simulink model "fuel_cell_tank"  (R2023a)
settings: Solver=VariableStepAuto  StartTime=0.0  StopTime=50  RelTol=1e-3
libraries: simulink x1
settings Model: Creator=connl  LastModifiedBy=connl

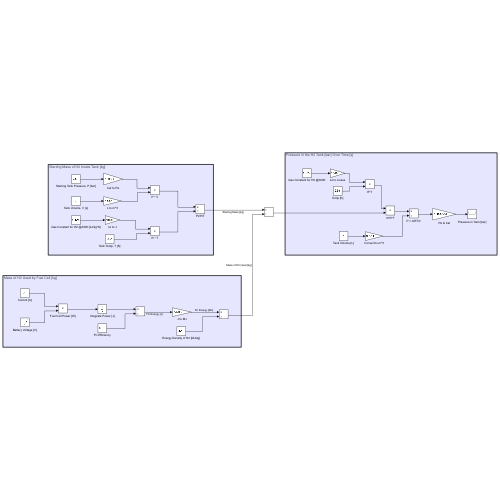
[thumbnail: Simulink's stored preview of the top-level diagram]
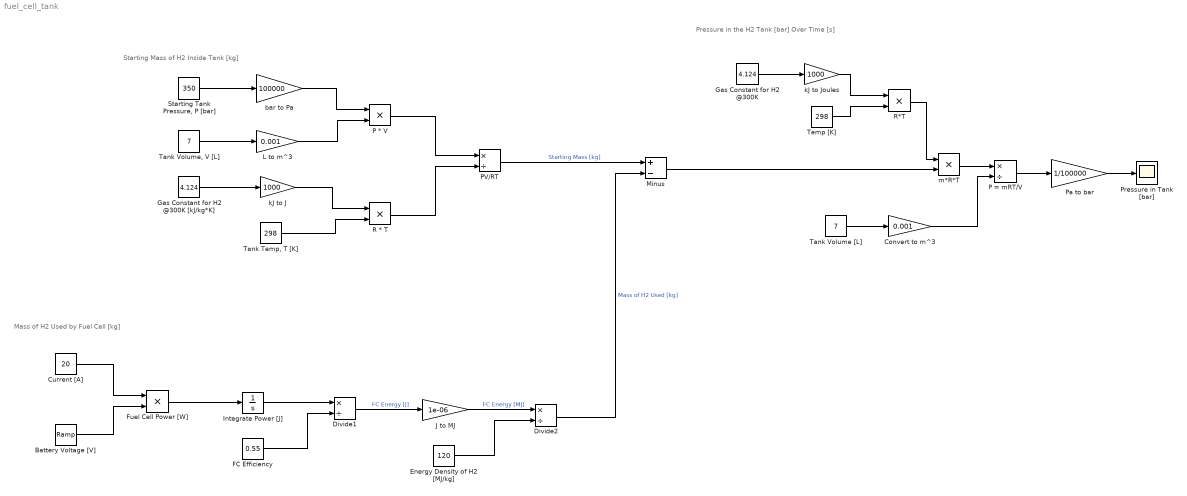
== system fuel_cell_tank ==
  note: Pressure in the H2 Tank [bar] Over Time [s]
  note: Mass of H2 Used by Fuel Cell [kg]
  note: Starting Mass of H2 Inside Tank [kg]
  Battery Voltage [V] : simulink/Sources/Ramp  slope=-1  start=0  InitialOutput=50
  Convert to m^3 : Gain  Gain=0.001
  Current [A] : Constant  Value=20
  Divide1 : Product  Inputs=*/
  Divide2 : Product  Inputs=*/
  Energy Density of H2 [MJ/kg] : Constant  Value=120
  FC Efficiency : Constant  Value=0.55
  Fuel Cell Power [W] : Product
  Gas Constant for H2 @300K : Constant  Value=4.124
  Gas Constant for H2 @300K [kJ/kg*K] : Constant  Value=4.124
  Integrate Power [J] : Integrator
  J to MJ : Gain  Gain=1e-06
  L to m^3 : Gain  Gain=0.001
  Minus : Sum  Inputs=+-
  P * V : Product
  P = mRT/V : Product  Inputs=*/
  PV/RT : Product  Inputs=*/
  Pa to bar : Gain  Gain=1/100000
  Pressure in Tank [bar] : Scope
  R * T : Product
  R*T : Product
  "Starting Tank Pressure, P [bar]" : Constant  Value=350
  "Tank Temp, T [K]" : Constant  Value=298
  Tank Volume [L] : Constant  Value=7
  "Tank Volume, V [L]" : Constant  Value=7
  Temp [K] : Constant  Value=298
  bar to Pa : Gain  Gain=100000
  kJ to J : Gain  Gain=1000
  kJ to Joules : Gain  Gain=1000
  m*R*T : Product
  wires:
  Integrate Power [J]/1 -> Divide1/1
  Divide2/1 -> Minus/2  "Mass of H2 Used [kg]"
  Fuel Cell Power [W]/1 -> Integrate Power [J]/1
  Current [A]/1 -> Fuel Cell Power [W]/1
  Battery Voltage [V]/1 -> Fuel Cell Power [W]/2
  Divide1/1 -> J to MJ/1  "FC Energy [J]"
  J to MJ/1 -> Divide2/1  "FC Energy [MJ]"
  bar to Pa/1 -> P * V/1
  FC Efficiency/1 -> Divide1/2
  Energy Density of H2 [MJ/kg]/1 -> Divide2/2
  "Starting Tank Pressure, P [bar]"/1 -> bar to Pa/1
  "Tank Volume, V [L]"/1 -> L to m^3/1
  L to m^3/1 -> P * V/2
  P * V/1 -> PV/RT/1
  "Tank Temp, T [K]"/1 -> R * T/2
  R * T/1 -> PV/RT/2
  Gas Constant for H2 @300K [kJ/kg*K]/1 -> kJ to J/1
  kJ to J/1 -> R * T/1
  PV/RT/1 -> Minus/1  "Starting Mass [kg]"
  Minus/1 -> m*R*T/2
  Gas Constant for H2 @300K/1 -> kJ to Joules/1
  Temp [K]/1 -> R*T/2
  R*T/1 -> m*R*T/1
  kJ to Joules/1 -> R*T/1
  m*R*T/1 -> P = mRT/V/1
  Tank Volume [L]/1 -> Convert to m^3/1
  Convert to m^3/1 -> P = mRT/V/2
  P = mRT/V/1 -> Pa to bar/1
  Pa to bar/1 -> Pressure in Tank [bar]/1
